simulink model "LAB1_InSIMULINK_MODULE"  (R2023a)
settings: Solver=VariableStepAuto  StartTime=0.0  StopTime=10.0  RelTol=1e-3
settings Model: Creator=alaam  LastModifiedBy=alaam

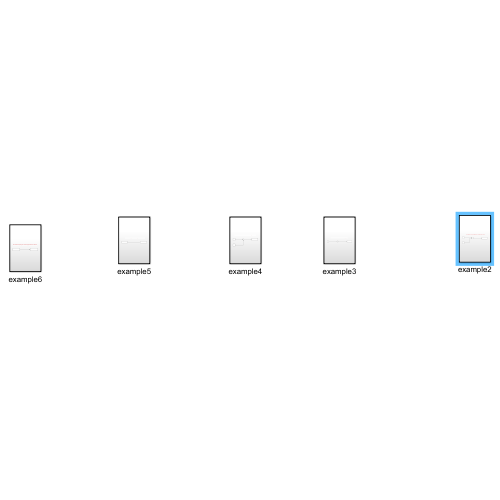
[thumbnail: Simulink's stored preview of the top-level diagram]
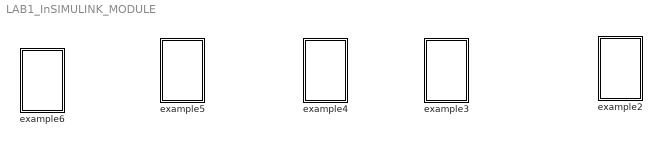
== system LAB1_InSIMULINK_MODULE ==
  example2 : Subsystem
  example3 : Subsystem
  example4 : Subsystem
  example5 : Subsystem
  example6 : Subsystem

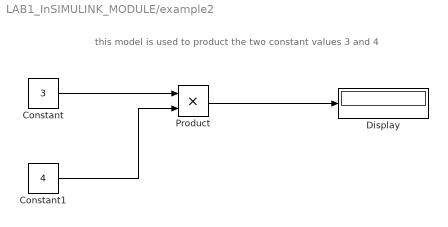
== system LAB1_InSIMULINK_MODULE/example2 ==
  note: this model is used to product the two constant values 3 and 4
  Constant : Constant  Value=3
  Constant1 : Constant  Value=4
  Display : Display
  Product : Product
  wires:
  Constant/1 -> Product/1
  Product/1 -> Display/1
  Constant1/1 -> Product/2

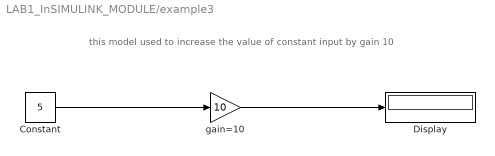
== system LAB1_InSIMULINK_MODULE/example3 ==
  note: this model used to increase the value of constant input by gain 10
  Constant : Constant  Value=5
  Display : Display
  gain=10 : Gain  Gain=10
  wires:
  gain=10/1 -> Display/1
  Constant/1 -> gain=10/1

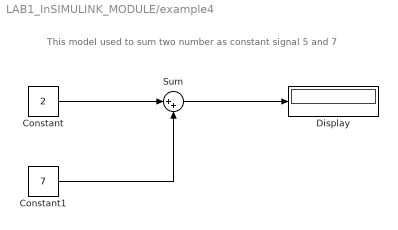
== system LAB1_InSIMULINK_MODULE/example4 ==
  note: This model used to sum two number as constant signal 5 and 7
  Constant : Constant  Value=2
  Constant1 : Constant  Value=7
  Display : Display
  Sum : Sum  Inputs=|++
  wires:
  Constant1/1 -> Sum/2
  Sum/1 -> Display/1
  Constant/1 -> Sum/1

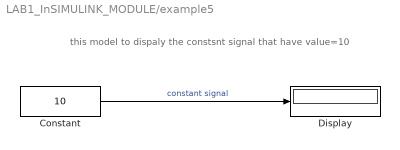
== system LAB1_InSIMULINK_MODULE/example5 ==
  note: this model to dispaly the constsnt signal that have value=10
  Constant : Constant  Value=10
  Display : Display
  wires:
  Constant/1 -> Display/1  "constant signal"

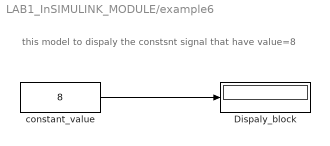
== system LAB1_InSIMULINK_MODULE/example6 ==
  note: this model to dispaly the constsnt signal that have value=8
  Dispaly_block : Display
  constant_value : Constant  Value=8
  wires:
  constant_value/1 -> Dispaly_block/1
